simulink model "EKF"  (R2020b)
settings: Solver=VariableStepAuto  StartTime=0.0  StopTime=tf  RelTol=1e-3
model workspace (MATLAB code in the model file):
  | %global Cv Ac Ts Fi_ss Qtrue
  | 
  | % Tank properties
  | Ac = 1.2; Cv = 0.8;
  | % Initial conditions
  | x0 = 1;
  | x1 = 1;
  | % Steady-state flow
  | Fi_ss = 2;
  | % Sampling interval
  | Ts = 0.1;
  | 
  | % Final time and time vector
  | tf = 127.4;
  | kvec = (0:Ts:tf)';
  | N = length(kvec);
  | 
  | % Input sequence (deviation from steady-state)
  | ukvec = idinput(N,'prbs',[0 0.2],[-1 1]);
  | simin = [kvec ukvec];
  | 
  | % Process and measurement noise covariances
  | Qtrue = [0.2 0; 0 0.1];
  | Rtrue = 0.1;
libraries: sharedTrackingLibrary x1
settings Model: OrderedModelArguments=off  Creator=arun  LastModifiedBy=prash

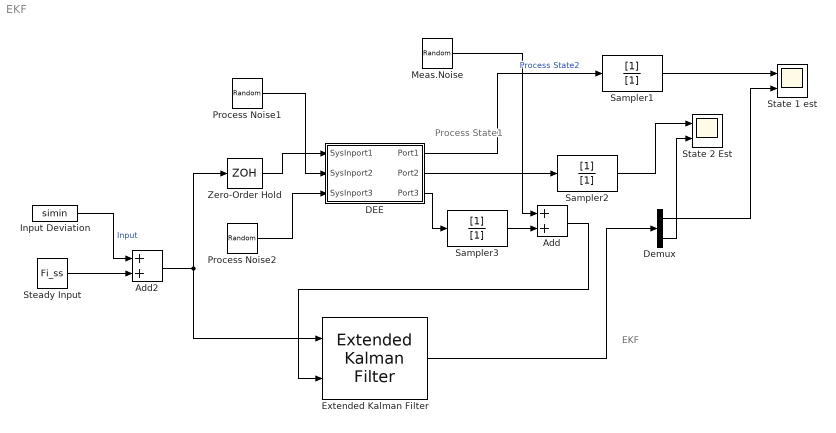
== system EKF ==
  note: Process
      | State1
  note: EKF
  Add : Sum
  Add2 : Sum
  DEE : Subsystem  mask(Differential Equation Editor (DEE)){}
      settings: OpenFcn=diffeqed
      mask Display: disp('Liquid Level \n System')
  Demux : Demux  Outputs=2
  Extended Kalman Filter : sharedTrackingLibrary/Extended Kalman Filter  StateTransitionFcn=liqlstatetrans_fun  HasStateTransitionJacobianFcn=off  HasAdditiveProcessNoise=Additive  ProcessNoise=Qtrue  HasTimeVaryingProcessNoise=off  HasStateTransitionFcnExtraArgument=1  InitialState=[1;1]  InitialStateCovariance=0.0001  MeasurementFcn1=liqlmeas_fun  HasMeasurementJacobianFcn1=off  HasMeasurementEnablePort1=off  HasAdditiveMeasurementNoise1=Additive  MeasurementNoise1=Rtrue  HasTimeVaryingMeasurementNoise1=off  HasMeasurementFcnExtraArgument1=0  MeasurementFcn2=myMeasurementFcn  HasMeasurementJacobianFcn2=off  HasMeasurementEnablePort2=off  HasAdditiveMeasurementNoise2=Additive  MeasurementNoise2=1  HasTimeVaryingMeasurementNoise2=off  HasMeasurementFcnExtraArgument2=0  MeasurementFcn3=myMeasurementFcn  HasMeasurementJacobianFcn3=off  HasMeasurementEnablePort3=off  HasAdditiveMeasurementNoise3=Additive  MeasurementNoise3=1  HasTimeVaryingMeasurementNoise3=off  HasMeasurementFcnExtraArgument3=0  MeasurementFcn4=myMeasurementFcn  HasMeasurementJacobianFcn4=off  HasMeasurementEnablePort4=off  HasAdditiveMeasurementNoise4=Additive  MeasurementNoise4=1  HasTimeVaryingMeasurementNoise4=off  HasMeasurementFcnExtraArgument4=0  MeasurementFcn5=myMeasurementFcn  HasMeasurementJacobianFcn5=off  HasMeasurementEnablePort5=off  HasAdditiveMeasurementNoise5=Additive  MeasurementNoise5=1  HasTimeVaryingMeasurementNoise5=off  HasMeasurementFcnExtraArgument5=0  EnableMultirate=off  StateTransitionFcnSampleTime=1  MeasurementFcn1SampleTime=1  MeasurementFcn2SampleTime=1  MeasurementFcn3SampleTime=1  MeasurementFcn4SampleTime=1  MeasurementFcn5SampleTime=1  UseCurrentEstimator=on  OutputStateCovariance=off  DataType=double  SampleTime=Ts  NumberOfMeasurements=1
      settings: SourceProductBaseCode=CT,DR,TF,ID,LP,NV,AR,RO,RR,UV,VE
  Input Deviation : FromWorkspace  VariableName=simin  SampleTime=Ts  Interpolate=off  OutputAfterFinalValue=Holding final value
  Meas.Noise : RandomNumber  Variance=Rtrue  Seed=4781  SampleTime=Ts
  Process Noise1 : RandomNumber  Variance=Qtrue(1,1)  Seed=38760  SampleTime=Ts
  Process Noise2 : RandomNumber  Variance=Qtrue(2,2)  Seed=4564  SampleTime=Ts
  Sampler1 : DiscreteFilter  Denominator=[1]  SampleTime=Ts
  Sampler2 : DiscreteFilter  Denominator=[1]  SampleTime=Ts
  Sampler3 : DiscreteFilter  Denominator=[1]  SampleTime=Ts
  State 1 est : Scope  NumInputPorts=2
  State 2 Est : Scope  NumInputPorts=2
  Steady Input : Constant  Value=Fi_ss  SampleTime=Ts
  Zero-Order Hold : ZeroOrderHold  SampleTime=Ts
  wires:
  Meas.Noise/1 -> Add/1
  Zero-Order Hold/1 -> DEE/1(SysInport1)
  Add/1 -> Extended Kalman Filter/2
  Extended Kalman Filter/1 -> Demux/1
  Steady Input/1 -> Add2/2
  Add2/1 -> Extended Kalman Filter/1, Zero-Order Hold/1
  Input Deviation/1 -> Add2/1  "Input"
  Sampler3/1 -> Add/2
  Process Noise1/1 -> DEE/2(SysInport2)
  Process Noise2/1 -> DEE/3(SysInport3)
  Demux/2 -> State 2 Est/2
  Sampler2/1 -> State 2 Est/1
  Sampler1/1 -> State 1 est/1
  Demux/1 -> State 1 est/2
  DEE/3(Port3) -> Sampler3/1
  DEE/2(Port2) -> Sampler2/1
  DEE/1(Port1) -> Sampler1/1  "Process State2"

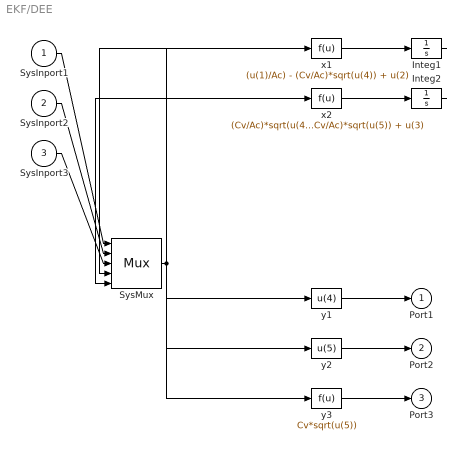
== system EKF/DEE ==
  SysInport1 : Inport
  SysInport2 : Inport  Port=2
  SysInport3 : Inport  Port=3
  Integ1 : Integrator  InitialCondition=x0
  Integ2 : Integrator  InitialCondition=x1
  SysMux : Mux  Inputs=5
  x1 : Fcn  Expr=(u(1)/Ac) - (Cv/Ac)*sqrt(u(4)) + u(2)
  x2 : Fcn  Expr=(Cv/Ac)*sqrt(u(4)) - (Cv/Ac)*sqrt(u(5)) + u(3)
  y1 : Fcn  Expr=u(4)
  y2 : Fcn  Expr=u(5)
  y3 : Fcn  Expr=Cv*sqrt(u(5))
  Port1 : Outport
  Port2 : Outport  Port=2
  Port3 : Outport  Port=3
  wires:
  SysInport1/1 -> SysMux/1
  SysInport2/1 -> SysMux/2
  SysInport3/1 -> SysMux/3
  SysMux/1 -> x1/1, x2/1, y1/1, y2/1, y3/1
  x1/1 -> Integ1/1
  Integ1/1 -> SysMux/4
  x2/1 -> Integ2/1
  Integ2/1 -> SysMux/5
  y1/1 -> Port1/1
  y2/1 -> Port2/1
  y3/1 -> Port3/1
